simulink model "pvBatteryManagement"  (R2023b)
settings: Solver=VariableStepAuto  StartTime=0.0  StopTime=10.0  RelTol=1e-3
undefined symbols (not defined in the file or in its folder): Acid, DiscIntNeverNeededParam, Lead
libraries: spsSeriesRLCBranchLib x7, spsVoltageMeasurementLib x5, spsCurrentMeasurementLib x4, spsIGBTDiodeLib x3, spsBatteryLib x1, spsBreakerLib x1, simulink x1, spsDiodeLib x1, spsPVArrayLib x1, spsPWMGeneratorDCDCLib x1, sps_lib x1
settings Model: Creator=Ashwin Soni  LastModifiedBy=Ashwin Soni

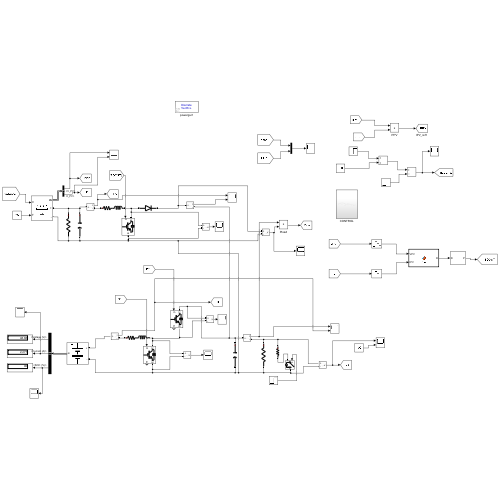
[thumbnail: Simulink's stored preview of the top-level diagram]
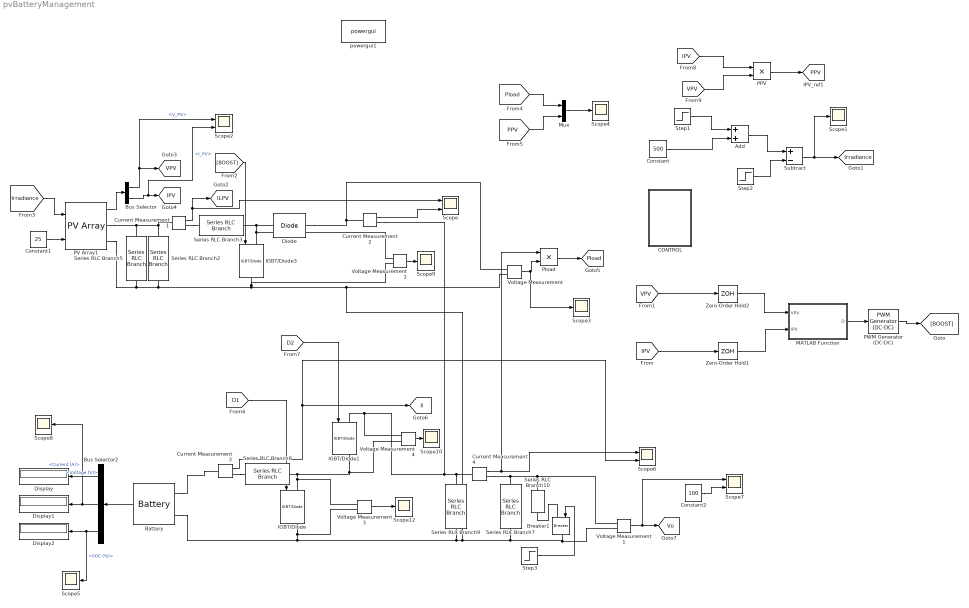
== system pvBatteryManagement ==
  Add : Sum
  Battery : spsBatteryLib/Battery  BatType=Lead-Acid  ShowTempParam=off  ThermalPreset=no  ShowAgeParam=off  NomV=48  NomQ=26  SOC=90  Batt_Tr=30  PresetModel=on  MaxQ=27.0833  MinV=36  FullV=52.2632  Dis_rate=5.2  R=0.018462  Normal_OP=8.0672  expZone="[48.8684    0.0866667]"  current=[6.5 13 32.5]  Units=Time  Tci=20  NomT=20  T2=-30  MaxQ2=4.8  FullV2=7.1  Normal_OP2=5.655  expZone2="[6.58           1]"  Rca=0.6  ti=2000  Dp=0  Neq0=0  Tsim=1e6  Ta1=25  Qeol=5.4*0.9  Reol=0.013333*1.2  Char_age=[2.3478, 3]  Dis_age=[2.3478, 10]  N1=1500  N2=10500  N3=1000  N4=1400  Ta2=45  N5=950
  Breaker1 : spsBreakerLib/Breaker  InitialState=0  SwitchingTimes="[1/60  5/60]"  External=on  BreakerResistance=0.01  SnubberResistance=1e6  SnubberCapacitance=inf  Measurements=None  MoreParameters=on  NoBreakLoop=off
  Bus Selector : BusSelector  OutputSignals=V_PV,I_PV
  Bus Selector2 : BusSelector  OutputSignals=Voltage (V),Current (A),SOC (%)
  CONTROL : Subsystem
  Constant : Constant  Value=500
  Constant1 : Constant  Value=25
  Constant2 : Constant  Value=100
  Current Measurement{1..4} (4 alike) : spsCurrentMeasurementLib/Current Measurement  PhasorSimulation=off  OutputType=Complex  PSBequivalent=0
  Diode : spsDiodeLib/Diode  Ron=0.001  Lon=0  Vf=0.8  IC=0  UseSnubber=0  Rs=inf  Cs=250e-9  Measurements=off
  Display : Display
  Display1 : Display
  Display2 : Display
  IGBT/Diode : spsIGBTDiodeLib/IGBT//Diode  Ron=1e-3  Rs=18  Cs=2.2e-6  Measurements=on
  IGBT/Diode1 : spsIGBTDiodeLib/IGBT//Diode  Ron=1e-3  Rs=18  Cs=2.2e-6  Measurements=on
  IGBT/Diode3 : spsIGBTDiodeLib/IGBT//Diode  Ron=1e-3  Rs=18  Cs=2.2e-6  Measurements=off
  MATLAB Function : MATLAB Function  TreatAsAtomicUnit=on
  Mux : Mux  Inputs=2
  PPV : Product
  PV Array1 : spsPVArrayLib/PV Array  Npar=2  Nser=2  PlotType=array @ 1000 W/m2 & specified temperatures  S_vec="[ 1000  500  100 ]"  Temp_C_vec="[ 45 25  ]"  ModuleName=Advance Solar Hydro Wind Power API-150  PlotWhenSelected=off  Pm=150.075  Ncell=72  Voc=41.8  Isc=5.05  Vm=34.5  Im=4.35  beta_Voc_pc=-0.419  alpha_Isc_pc=0.096  beta_Voc=-0.17514  alpha_Isc=0.004848  IL=5.0762  I0=1.155e-09  nI=1.0233  Rsh=71.9537  Rs=0.37337  RobustModel=off  RobustCellTemperature=313.3991  BAL=on  Tc=1e-6  Tfilter=5e-5
  PWM Generator (DC-DC) : spsPWMGeneratorDCDCLib/PWM Generator (DC-DC)  Fsw=10000  Ts=0
  Pload : Product
  Scope{,2,6..7} (4 alike) : Scope  NumInputPorts=2
  Scope{1,3..5,8..10,12} (8 alike) : Scope
  Series RLC Branch10 : spsSeriesRLCBranchLib/Series RLC Branch  LConnTagsString=__new0  RConnTagsString=__new0  BranchType=R  Resistance=500  Inductance=10e-3  SetiL0=off  InitialCurrent=0  Capacitance=1e-6  Setx0=off  InitialVoltage=0  Measurements=None
  Series RLC Branch2 : spsSeriesRLCBranchLib/Series RLC Branch  LConnTagsString=__new0  RConnTagsString=__new0  BranchType=C  Resistance=1  Inductance=1e-3  SetiL0=off  InitialCurrent=0  Capacitance=47e-6  Setx0=off  InitialVoltage=0  Measurements=None
  Series RLC Branch3 : spsSeriesRLCBranchLib/Series RLC Branch  LConnTagsString=__new0  RConnTagsString=__new0  BranchType=RL  Resistance=1  Inductance=6.4e-3  SetiL0=off  InitialCurrent=0  Capacitance=1e-6  Setx0=off  InitialVoltage=0  Measurements=None
  Series RLC Branch5 : spsSeriesRLCBranchLib/Series RLC Branch  LConnTagsString=__new0  RConnTagsString=__new0  BranchType=R  Resistance=10E6  Inductance=10e-3  SetiL0=off  InitialCurrent=0  Capacitance=1e-6  Setx0=off  InitialVoltage=0  Measurements=None
  Series RLC Branch7 : spsSeriesRLCBranchLib/Series RLC Branch  LConnTagsString=__new0  RConnTagsString=__new0  BranchType=R  Resistance=500  Inductance=10e-3  SetiL0=off  InitialCurrent=0  Capacitance=1e-6  Setx0=off  InitialVoltage=0  Measurements=None
  Series RLC Branch8 : spsSeriesRLCBranchLib/Series RLC Branch  LConnTagsString=__new0  RConnTagsString=__new0  BranchType=RL  Resistance=1  Inductance=6.4e-3  SetiL0=off  InitialCurrent=0  Capacitance=1e-6  Setx0=off  InitialVoltage=0  Measurements=None
  Series RLC Branch9 : spsSeriesRLCBranchLib/Series RLC Branch  LConnTagsString=__new0  RConnTagsString=__new0  BranchType=C  Resistance=1  Inductance=1e-3  SetiL0=off  InitialCurrent=0  Capacitance=100e-6  Setx0=off  InitialVoltage=0  Measurements=None
  Step1 : Step  Time=3  After=300  SampleTime=0
  Step2 : Step  Time=8  After=300  SampleTime=0
  Step3 : Step  Time=5  SampleTime=0
  Subtract : Sum  Inputs=+-
  Voltage Measurement{,1..4} (5 alike) : spsVoltageMeasurementLib/Voltage Measurement  PhasorSimulation=off  OutputType=Complex  PSBequivalent=0
  Zero-Order Hold1 : ZeroOrderHold  SampleTime=50e-4
  Zero-Order Hold2 : ZeroOrderHold  SampleTime=50e-4
  powergui1 : sps_lib/powergui  Priority=1  SimulationMode=Discrete  SampleTime=5e-6  frequency=60  Iterations=50  frequencyindice=0  Pbase=100e6  ErrMax=1e-4  UnitsV=kV  UnitsW=MW  buscounter=0  FunctionMessages=off  echomessages=off  EnableUseOfTLC=off  CurrentSourceSwitches=off  DisableSnubberDevices=off  DisableRonSwitches=off  DisableVfSwitches=off  DisplayEquations=off  AutomaticDiscreteSolvers=off  SolverType=Tustin/Backward Euler (TBE)  Interpol=off  ExternalGateDelay=off  methode=off  Ts=100  x0status=blocks  SPID=on  SwTol=0  HookPort=off  NonlinearTolerance=1e-4  nMaxIteration=100  ContinueOnMaxIteration=off  RestoreLinks=warning  ResistiveCurrentMeasurement=off  Frange=[0:2:500]  Ylog=off  Xlog=on  ShowGrid=off  save=off  variable=ZData  structure=0  ZoomFFT=off  StartTime=0.0  cycles=1  DisplayStyle=1  fundamental=60  FreqAxis=off  MaxFrequency=1000  frequencyindicesteady=1  RmsSteady=1  display=off
  tag scope: ILPV=global, IPV=global, Il=global, Irradiance=global, PPV=global, Pload=global, VPV=global, Vo=global
  wires:
  Voltage Measurement4/1 -> Scope10/1
  Voltage Measurement2/1 -> Scope9/1
  Voltage Measurement3/1 -> Scope12/1
  [VPV] -> PPV/2
  Bus Selector2/3 -> Scope5/1, Display2/1  "<SOC (%)>"
  Mux/1 -> Scope4/1
  Bus Selector2/2 -> Scope8/1, Display1/1  "<Current (A)>"
  Voltage Measurement1/1 -> Scope7/1, [Vo]
  [IPV] -> PPV/1
  [VPV] -> Zero-Order Hold2/1
  Step1/1 -> Add/1
  Battery/1 -> Bus Selector2/1
  Bus Selector2/1 -> Display/1  "<Voltage (V)>"
  PWM Generator (DC-DC)/1 -> [BOOST]
  Current Measurement4/1 -> Pload/1, Scope6/1
  PPV/1 -> [PPV]
  Step3/1 -> Breaker1/1
  [D2] -> IGBT/Diode1/1
  Current Measurement3/1 -> [Il], Scope6/2
  Constant2/1 -> Scope7/2
  Bus Selector/1 -> Scope2/1, [VPV]  "<V_PV>"
  Current Measurement2/1 -> Scope/2
  [PPV] -> Mux/2
  Constant1/1 -> PV Array1/2
  Current Measurement1/1 -> Scope/1, [ILPV]
  [IPV] -> Zero-Order Hold1/1
  Voltage Measurement/1 -> Scope3/1, Pload/2
  PV Array1/1 -> Bus Selector/1
  MATLAB Function/1(D) -> PWM Generator (DC-DC)/1
  Bus Selector/2 -> Scope2/2, [IPV]  "<I_PV>"
  [BOOST] -> IGBT/Diode3/1
  Constant/1 -> Add/2
  Add/1 -> Subtract/1
  Zero-Order Hold2/1 -> MATLAB Function/1(VPV)
  Subtract/1 -> Scope1/1, [Irradiance]
  Pload/1 -> [Pload]
  [Pload] -> Mux/1
  Step2/1 -> Subtract/2
  Zero-Order Hold1/1 -> MATLAB Function/2(IPV)
  [Irradiance] -> PV Array1/1
  [D1] -> IGBT/Diode/1
  connections:
  Voltage Measurement/LConn1 -- Diode/RConn1 -- Current Measurement2/LConn1
  PV Array1/RConn2 -- IGBT/Diode3/RConn1 -- Voltage Measurement2/LConn2 -- Voltage Measurement1/LConn2 -- Breaker1/RConn1 -- Series RLC Branch7/RConn1 -- Voltage Measurement3/LConn2 -- IGBT/Diode/RConn1 -- Battery/LConn2 -- Series RLC Branch9/RConn1 -- Voltage Measurement/LConn2 -- Series RLC Branch2/RConn1 -- Series RLC Branch5/RConn1
  Series RLC Branch9/LConn1 -- Current Measurement4/LConn1 -- Current Measurement2/RConn1 -- IGBT/Diode1/LConn1 -- Voltage Measurement4/LConn1
  Voltage Measurement4/LConn2 -- Series RLC Branch8/RConn1 -- Voltage Measurement3/LConn1 -- IGBT/Diode/LConn1 -- IGBT/Diode1/RConn1
  Series RLC Branch2/LConn1 -- Current Measurement1/LConn1 -- PV Array1/RConn1 -- Series RLC Branch5/LConn1
  Series RLC Branch7/LConn1 -- Voltage Measurement1/LConn1 -- Series RLC Branch10/LConn1 -- Current Measurement4/RConn1
  Voltage Measurement2/LConn1 -- Series RLC Branch3/RConn1 -- Diode/LConn1 -- IGBT/Diode3/LConn1
  Current Measurement3/RConn1 -- Series RLC Branch8/LConn1
  Battery/LConn1 -- Current Measurement3/LConn1
  Current Measurement1/RConn1 -- Series RLC Branch3/LConn1
  Breaker1/LConn1 -- Series RLC Branch10/RConn1

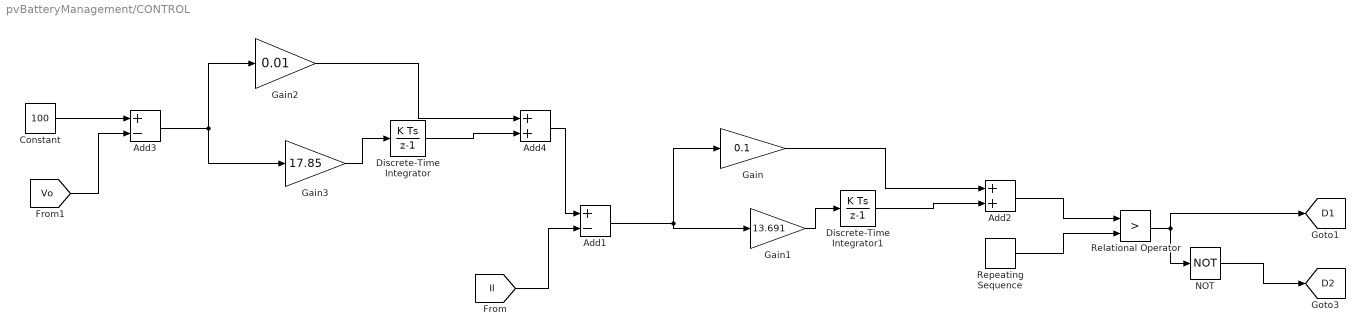
== system pvBatteryManagement/CONTROL ==
  Add1 : Sum  Inputs=+-
  Add2 : Sum
  Add3 : Sum  Inputs=+-
  Add4 : Sum
  Constant : Constant  Value=100
  Discrete-Time Integrator : DiscreteIntegrator  SampleTime=-1  ICPrevOutput=DiscIntNeverNeededParam  ICPrevScaledInput=DiscIntNeverNeededParam
  Discrete-Time Integrator1 : DiscreteIntegrator  SampleTime=-1  ICPrevOutput=DiscIntNeverNeededParam  ICPrevScaledInput=DiscIntNeverNeededParam
  Gain : Gain  Gain=0.1
  Gain1 : Gain  Gain=13.691
  Gain2 : Gain  Gain=0.01
  Gain3 : Gain  Gain=17.85
  NOT : Logic  Operator=NOT  IconShape=distinctive  AllPortsSameDT=off  OutDataTypeStr=boolean
  Relational Operator : RelationalOperator  Operator=>  OutDataTypeStr=boolean  RndMeth=Simplest  InputSameDT=off
  Repeating Sequence : simulink/Sources/Repeating Sequence  rep_seq_t=[0 0.5 1]*(1/(10e3))  rep_seq_y=[0 1 0]
  tag scope: D1=global, D2=global
  wires:
  NOT/1 -> [D2]
  [Il] -> Add1/2
  Gain/1 -> Add2/1
  Add1/1 -> Gain/1, Gain1/1
  Add2/1 -> Relational Operator/1
  Discrete-Time Integrator1/1 -> Add2/2
  Relational Operator/1 -> NOT/1, [D1]
  Gain1/1 -> Discrete-Time Integrator1/1
  Repeating Sequence/1 -> Relational Operator/2
  Gain3/1 -> Discrete-Time Integrator/1
  Discrete-Time Integrator/1 -> Add4/2
  Add3/1 -> Gain2/1, Gain3/1
  Gain2/1 -> Add4/1
  [Vo] -> Add3/2
  Add4/1 -> Add1/1
  Constant/1 -> Add3/1

== matlab function pvBatteryManagement/MATLAB Function ==
  data: VPV input; D output; IPV input
function D = fcn(VPV,IPV)

% f = 100000hz (G)

Dinit = 0.5; %Initial value for D output
Dmax = 0.99; %Maximum value for D
Dmin = 0.1; %Minimum value for D
deltaD = 0.005; %Increment value used to increae/decrease the duty cycle D

persistent Vold Pold Dold M Iold;

dataType = 'double';

 if isempty(Vold)
     Vold=0;
     Pold=0;
     Iold=0;
     Dold=Dinit;
     M=1;
 end
 PPV = VPV*IPV;
 dVPV = VPV - Vold;
 dPPV = PPV - Pold;
 dIPV = IPV - Iold;
 M=1;
 if M <0.005
     D=Dold;
 else
     if dVPV == 0
         if dIPV == 0
             D=Dold;
         elseif dIPV>0
             D=Dold - (M*deltaD);
         else
             D=Dold + (M*deltaD);
         end
     else
         if dIPV/dVPV == -IPV/VPV
             D=Dold;
         elseif dIPV/dVPV>-IPV/VPV
             D=Dold - (M*deltaD);
         else
             D=Dold + (M*deltaD);
         end
     end
 end
 
 if D>=Dmax || D<=Dmin
     D=Dold;
 end
 
 Dold=D;
 Vold=VPV;
 Pold=PPV;
 Iold=IPV;
